simulink model "AerodynamicsSinglePlateHarness"  (R2025a)
settings: Solver=FixedStepDiscrete  StartTime=0  StopTime=200  FixedStep=1  RelTol=1e-09  AbsTol=1e-10
settings Model: Creator=juliankazmierski  LastModifiedBy=juliankazmierski

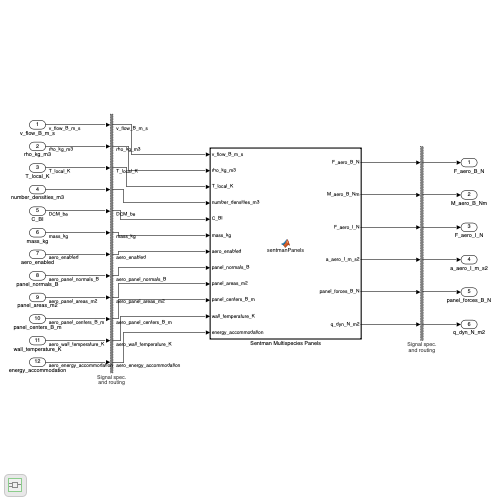
[thumbnail: Simulink's stored preview of the top-level diagram]
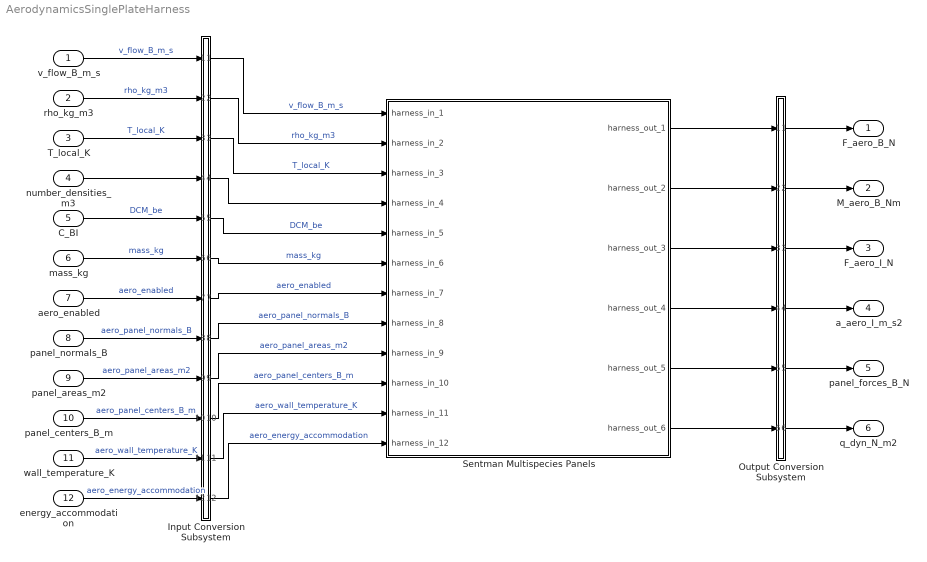
== system AerodynamicsSinglePlateHarness ==
  v_flow_B_m_s : Inport  OutDataTypeStr=double  PortDimensions=[3, 1]  SampleTime=0
  rho_kg_m3 : Inport  Port=2  OutDataTypeStr=double  PortDimensions=[1]  SampleTime=0
  T_local_K : Inport  Port=3  OutDataTypeStr=double  PortDimensions=[1]  SampleTime=0
  number_densities_m3 : Inport  Port=4  OutDataTypeStr=double  PortDimensions=[6]  SampleTime=0
  C_BI : Inport  Port=5  OutDataTypeStr=double  PortDimensions=[3, 3]  SampleTime=0
  mass_kg : Inport  Port=6  OutDataTypeStr=double  PortDimensions=[1]  SampleTime=[-1, 0]
  aero_enabled : Inport  Port=7  OutDataTypeStr=double  PortDimensions=[1]  SampleTime=[-1, 0]
  panel_normals_B : Inport  Port=8  OutDataTypeStr=double  PortDimensions=[3, 6]  SampleTime=[-1, 0]
  panel_areas_m2 : Inport  Port=9  OutDataTypeStr=double  PortDimensions=[6, 1]  SampleTime=[-1, 0]
  panel_centers_B_m : Inport  Port=10  OutDataTypeStr=double  PortDimensions=[3, 6]  SampleTime=[-1, 0]
  wall_temperature_K : Inport  Port=11  OutDataTypeStr=double  PortDimensions=[6, 1]  SampleTime=[-1, 0]
  energy_accommodation : Inport  Port=12  OutDataTypeStr=double  PortDimensions=[6, 1]  SampleTime=[-1, 0]
  Input Conversion Subsystem : Subsystem  Tag=__SLT_ICS__  Description=|
      | Signal spec.
      | and routing
      settings: AttributesFormatString=%<Description>
  Output Conversion Subsystem : Subsystem  Tag=__SLT_OCS__  Description=|
      | Signal spec.
      | and routing
      settings: AttributesFormatString=%<Description>
  Sentman Multispecies Panels : Subsystem  Tag=__SL_testing_harness_stub_
  F_aero_B_N : Outport
  M_aero_B_Nm : Outport  Port=2
  F_aero_I_N : Outport  Port=3
  a_aero_I_m_s2 : Outport  Port=4
  panel_forces_B_N : Outport  Port=5
  q_dyn_N_m2 : Outport  Port=6
  wires:
  v_flow_B_m_s/1 -> Input Conversion Subsystem/1(Inport_1)  "v_flow_B_m_s"
  rho_kg_m3/1 -> Input Conversion Subsystem/2(Inport_2)  "rho_kg_m3"
  T_local_K/1 -> Input Conversion Subsystem/3(Inport_3)  "T_local_K"
  number_densities_m3/1 -> Input Conversion Subsystem/4(Inport_4)
  C_BI/1 -> Input Conversion Subsystem/5(Inport_5)  "DCM_be"
  mass_kg/1 -> Input Conversion Subsystem/6(Inport_6)  "mass_kg"
  aero_enabled/1 -> Input Conversion Subsystem/7(Inport_7)  "aero_enabled"
  panel_normals_B/1 -> Input Conversion Subsystem/8(Inport_8)  "aero_panel_normals_B"
  panel_areas_m2/1 -> Input Conversion Subsystem/9(Inport_9)  "aero_panel_areas_m2"
  panel_centers_B_m/1 -> Input Conversion Subsystem/10(Inport_10)  "aero_panel_centers_B_m"
  wall_temperature_K/1 -> Input Conversion Subsystem/11(Inport_11)  "aero_wall_temperature_K"
  energy_accommodation/1 -> Input Conversion Subsystem/12(Inport_12)  "aero_energy_accommodation"
  Output Conversion Subsystem/1(Outport_1) -> F_aero_B_N/1
  Output Conversion Subsystem/2(Outport_2) -> M_aero_B_Nm/1
  Output Conversion Subsystem/3(Outport_3) -> F_aero_I_N/1
  Output Conversion Subsystem/4(Outport_4) -> a_aero_I_m_s2/1
  Output Conversion Subsystem/5(Outport_5) -> panel_forces_B_N/1
  Output Conversion Subsystem/6(Outport_6) -> q_dyn_N_m2/1
  Input Conversion Subsystem/1(Outport_1) -> Sentman Multispecies Panels/1(harness_in_1)  "v_flow_B_m_s"
  Input Conversion Subsystem/2(Outport_2) -> Sentman Multispecies Panels/2(harness_in_2)  "rho_kg_m3"
  Input Conversion Subsystem/3(Outport_3) -> Sentman Multispecies Panels/3(harness_in_3)  "T_local_K"
  Input Conversion Subsystem/4(Outport_4) -> Sentman Multispecies Panels/4(harness_in_4)
  Input Conversion Subsystem/5(Outport_5) -> Sentman Multispecies Panels/5(harness_in_5)  "DCM_be"
  Input Conversion Subsystem/6(Outport_6) -> Sentman Multispecies Panels/6(harness_in_6)  "mass_kg"
  Input Conversion Subsystem/7(Outport_7) -> Sentman Multispecies Panels/7(harness_in_7)  "aero_enabled"
  Input Conversion Subsystem/8(Outport_8) -> Sentman Multispecies Panels/8(harness_in_8)  "aero_panel_normals_B"
  Input Conversion Subsystem/9(Outport_9) -> Sentman Multispecies Panels/9(harness_in_9)  "aero_panel_areas_m2"
  Input Conversion Subsystem/10(Outport_10) -> Sentman Multispecies Panels/10(harness_in_10)  "aero_panel_centers_B_m"
  Input Conversion Subsystem/11(Outport_11) -> Sentman Multispecies Panels/11(harness_in_11)  "aero_wall_temperature_K"
  Input Conversion Subsystem/12(Outport_12) -> Sentman Multispecies Panels/12(harness_in_12)  "aero_energy_accommodation"
  Sentman Multispecies Panels/1(harness_out_1) -> Output Conversion Subsystem/1(Inport_1)
  Sentman Multispecies Panels/2(harness_out_2) -> Output Conversion Subsystem/2(Inport_2)
  Sentman Multispecies Panels/3(harness_out_3) -> Output Conversion Subsystem/3(Inport_3)
  Sentman Multispecies Panels/4(harness_out_4) -> Output Conversion Subsystem/4(Inport_4)
  Sentman Multispecies Panels/5(harness_out_5) -> Output Conversion Subsystem/5(Inport_5)
  Sentman Multispecies Panels/6(harness_out_6) -> Output Conversion Subsystem/6(Inport_6)

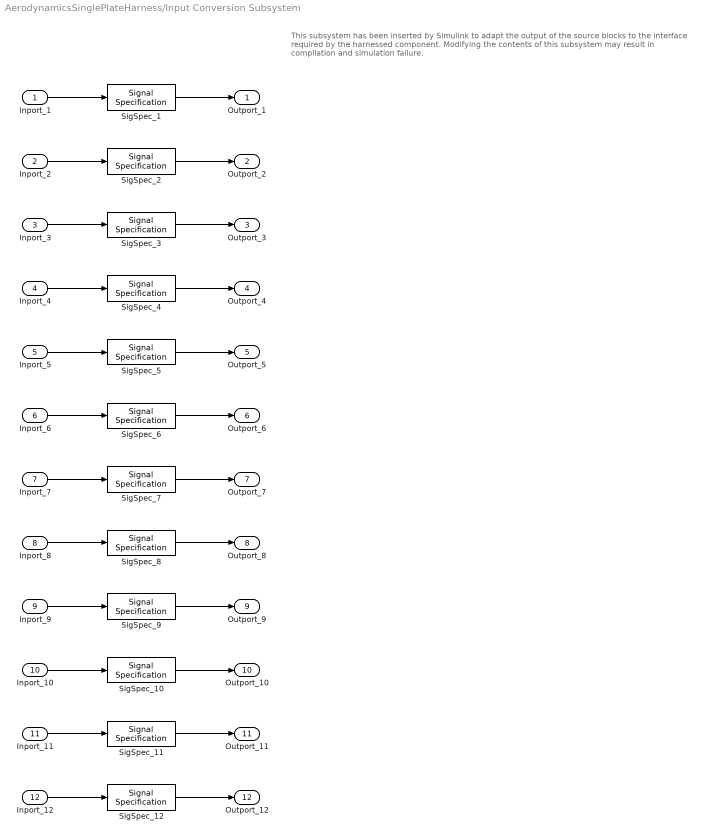
== system AerodynamicsSinglePlateHarness/Input Conversion Subsystem ==
  note: This subsystem has been inserted by Simulink to adapt the output of the source blocks to the interface required by the harnessed component.
      |  Modifying the contents of this subsystem may result in compilation and simulation failure.
  Inport_1 : Inport
  Inport_2 : Inport  Port=2
  Inport_3 : Inport  Port=3
  Inport_4 : Inport  Port=4
  Inport_5 : Inport  Port=5
  Inport_6 : Inport  Port=6
  Inport_7 : Inport  Port=7
  Inport_8 : Inport  Port=8
  Inport_9 : Inport  Port=9
  Inport_10 : Inport  Port=10
  Inport_11 : Inport  Port=11
  Inport_12 : Inport  Port=12
  SigSpec_1 : SignalSpecification  OutDataTypeStr=double  Dimensions=[3, 1]  SampleTime=[0, 0]
  SigSpec_10 : SignalSpecification  OutDataTypeStr=double  Unit=m  Dimensions=[3, 6]  SampleTime=[-1, 0]
  SigSpec_11 : SignalSpecification  OutDataTypeStr=double  Unit=K  Dimensions=[6, 1]  SampleTime=[-1, 0]
  SigSpec_12 : SignalSpecification  OutDataTypeStr=double  Unit=1  Dimensions=[6, 1]  SampleTime=[-1, 0]
  SigSpec_2 : SignalSpecification  OutDataTypeStr=double  Unit=kg/m^3  Dimensions=[1]  SampleTime=[0, 0]
  SigSpec_3 : SignalSpecification  OutDataTypeStr=double  Unit=K  Dimensions=[1]  SampleTime=[0, 0]
  SigSpec_4 : SignalSpecification  OutDataTypeStr=double  Unit=1/m^3  Dimensions=[6]  SampleTime=[0, 0]
  SigSpec_5 : SignalSpecification  OutDataTypeStr=double  Unit=1  Dimensions=[3, 3]  SampleTime=[0, 0]
  SigSpec_6 : SignalSpecification  OutDataTypeStr=double  Unit=kg  Dimensions=[1]  SampleTime=[-1, 0]
  SigSpec_7 : SignalSpecification  OutDataTypeStr=double  Unit=1  Dimensions=[1]  SampleTime=[-1, 0]
  SigSpec_8 : SignalSpecification  OutDataTypeStr=double  Unit=1  Dimensions=[3, 6]  SampleTime=[-1, 0]
  SigSpec_9 : SignalSpecification  OutDataTypeStr=double  Unit=m^2  Dimensions=[6, 1]  SampleTime=[-1, 0]
  Outport_1 : Outport
  Outport_2 : Outport  Port=2
  Outport_3 : Outport  Port=3
  Outport_4 : Outport  Port=4
  Outport_5 : Outport  Port=5
  Outport_6 : Outport  Port=6
  Outport_7 : Outport  Port=7
  Outport_8 : Outport  Port=8
  Outport_9 : Outport  Port=9
  Outport_10 : Outport  Port=10
  Outport_11 : Outport  Port=11
  Outport_12 : Outport  Port=12
  wires:
  SigSpec_1/1 -> Outport_1/1
  Inport_1/1 -> SigSpec_1/1
  SigSpec_2/1 -> Outport_2/1
  Inport_2/1 -> SigSpec_2/1
  SigSpec_3/1 -> Outport_3/1
  Inport_3/1 -> SigSpec_3/1
  SigSpec_4/1 -> Outport_4/1
  Inport_4/1 -> SigSpec_4/1
  SigSpec_5/1 -> Outport_5/1
  Inport_5/1 -> SigSpec_5/1
  SigSpec_6/1 -> Outport_6/1
  Inport_6/1 -> SigSpec_6/1
  SigSpec_7/1 -> Outport_7/1
  Inport_7/1 -> SigSpec_7/1
  SigSpec_8/1 -> Outport_8/1
  Inport_8/1 -> SigSpec_8/1
  SigSpec_9/1 -> Outport_9/1
  Inport_9/1 -> SigSpec_9/1
  SigSpec_10/1 -> Outport_10/1
  Inport_10/1 -> SigSpec_10/1
  SigSpec_11/1 -> Outport_11/1
  Inport_11/1 -> SigSpec_11/1
  SigSpec_12/1 -> Outport_12/1
  Inport_12/1 -> SigSpec_12/1

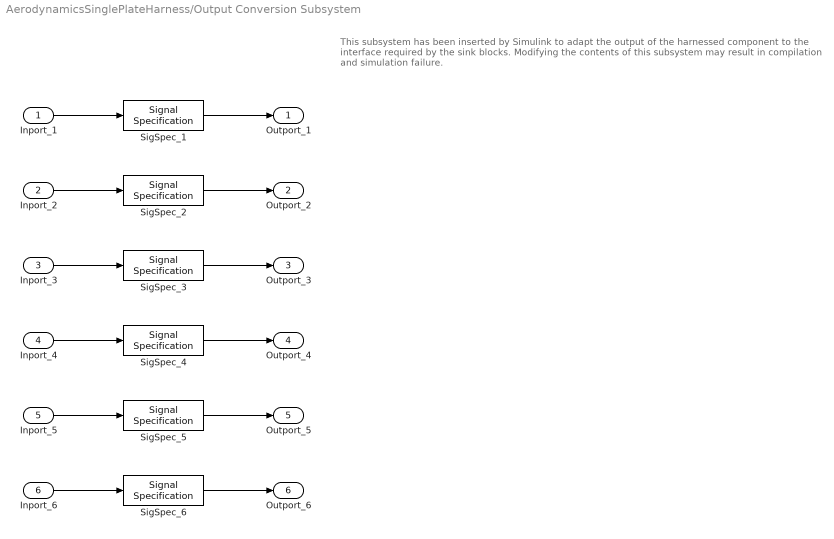
== system AerodynamicsSinglePlateHarness/Output Conversion Subsystem ==
  note: This subsystem has been inserted by Simulink to adapt the output of the harnessed component to the interface required by the sink blocks.
      |  Modifying the contents of this subsystem may result in compilation and simulation failure.
  Inport_1 : Inport
  Inport_2 : Inport  Port=2
  Inport_3 : Inport  Port=3
  Inport_4 : Inport  Port=4
  Inport_5 : Inport  Port=5
  Inport_6 : Inport  Port=6
  SigSpec_1 : SignalSpecification  OutDataTypeStr=double  Dimensions=[3, 1]
  SigSpec_2 : SignalSpecification  OutDataTypeStr=double  Dimensions=[3, 1]
  SigSpec_3 : SignalSpecification  OutDataTypeStr=double  Dimensions=[3, 1]
  SigSpec_4 : SignalSpecification  OutDataTypeStr=double  Unit=m/s^2  Dimensions=[3, 1]
  SigSpec_5 : SignalSpecification  OutDataTypeStr=double  Dimensions=[3, 6]
  SigSpec_6 : SignalSpecification  OutDataTypeStr=double  Dimensions=[1]
  Outport_1 : Outport
  Outport_2 : Outport  Port=2
  Outport_3 : Outport  Port=3
  Outport_4 : Outport  Port=4
  Outport_5 : Outport  Port=5
  Outport_6 : Outport  Port=6
  wires:
  Inport_1/1 -> SigSpec_1/1
  SigSpec_1/1 -> Outport_1/1
  Inport_2/1 -> SigSpec_2/1
  SigSpec_2/1 -> Outport_2/1
  Inport_3/1 -> SigSpec_3/1
  SigSpec_3/1 -> Outport_3/1
  Inport_4/1 -> SigSpec_4/1
  SigSpec_4/1 -> Outport_4/1
  Inport_5/1 -> SigSpec_5/1
  SigSpec_5/1 -> Outport_5/1
  Inport_6/1 -> SigSpec_6/1
  SigSpec_6/1 -> Outport_6/1

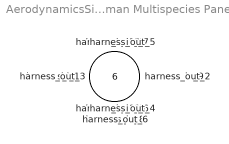
== system AerodynamicsSinglePlateHarness/Sentman Multispecies Panels ==
  harness_in_1 : Inport
  harness_in_2 : Inport  Port=2
  harness_in_3 : Inport  Port=3
  harness_in_4 : Inport  Port=4
  harness_in_5 : Inport  Port=5
  harness_in_6 : Inport  Port=6
  harness_in_7 : Inport  Port=7
  harness_in_8 : Inport  Port=8
  harness_in_9 : Inport  Port=9
  harness_in_10 : Inport  Port=10
  harness_in_11 : Inport  Port=11
  harness_in_12 : Inport  Port=12
  harness_out_1 : Outport
  harness_out_2 : Outport  Port=2
  harness_out_3 : Outport  Port=3
  harness_out_4 : Outport  Port=4
  harness_out_5 : Outport  Port=5
  harness_out_6 : Outport  Port=6
